simulink model "asr_ut"  (Simulink 8.1)
settings: Solver=FixedStepDiscrete  StartTime=0.0  StopTime=10.0  FixedStep=5E-3  RelTol=1e-3
libraries: siltestlib x2, asr x1
settings Model: Creator=AT015086  LastModifiedBy=AT015086
settings DataIOCC: SignalLoggingSaveFormat=Dataset
settings OptimizationCC: ExpressionDepthLimit=128
settings DebuggingCC: FcnCallInpInsideContextMsg=EnableAllAsError
settings GRTTargetCC: CombineOutputUpdateFcns=on  GRTInterface=off

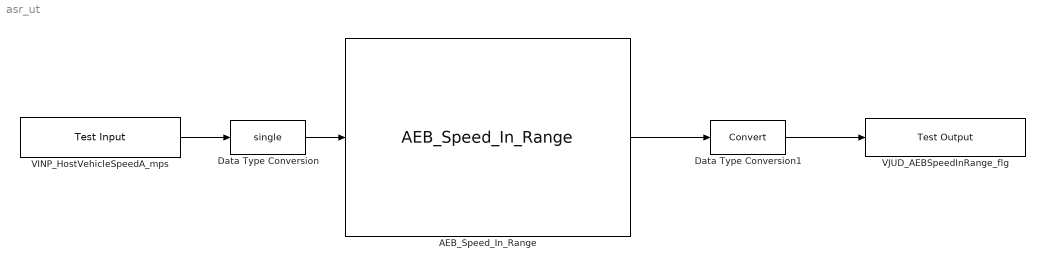
== system asr_ut ==
  AEB_Speed_In_Range : asr/AEB_Speed_In_Range
  Data Type Conversion : DataTypeConversion  OutDataTypeStr=single
  Data Type Conversion1 : DataTypeConversion
  VINP_HostVehicleSpeedA_mps : siltestlib/Test Input  varname=VINP_HostVehicleSpeedA_mps  sampletime=-1
  VJUD_AEBSpeedInRange_flg : siltestlib/Test Output  varname=VJUD_AEBSpeedInRange_flg  sampletime=-1
  wires:
  VINP_HostVehicleSpeedA_mps/1 -> Data Type Conversion/1
  Data Type Conversion/1 -> AEB_Speed_In_Range/1
  AEB_Speed_In_Range/1 -> Data Type Conversion1/1
  Data Type Conversion1/1 -> VJUD_AEBSpeedInRange_flg/1
